simulink model "Modelo_Red_Mitigación_final"  (R2019b)
settings: Solver=VariableStepAuto  StartTime=0.0  StopTime=2.5  RelTol=1e-3
InitFcn:
  | Ts=20e-6;
undefined symbols (not defined in the file): D1, Delta, Ion, Lithium
libraries: powerlib x371, powerlib_meascontrol x286, simulink x50, simulink_extras x20, electricdrivelib x16
(part 2 of 11)

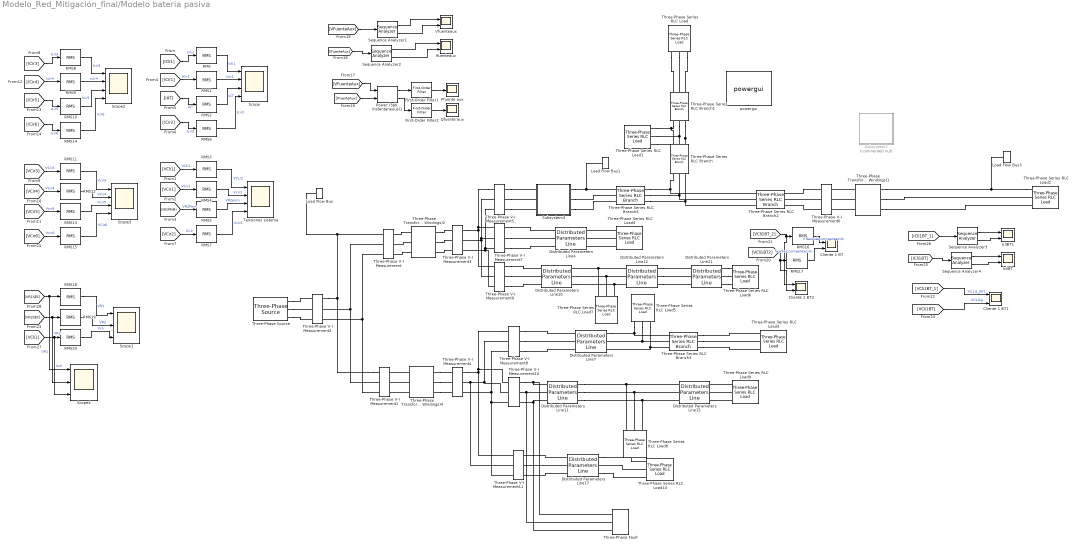
== system Modelo_Red_Mitigación_final/Modelo bateria pasiva ==
  Cliente 1 BT : Scope  NumInputPorts=2
  Cliente 1 BT1 : Scope  NumInputPorts=3
  Cliente 1 BT2 : Scope  NumInputPorts=2
  Distributed Parameters Line10 : powerlib/Elements/Distributed Parameters Line  Phases=3  Frequency=60  Resistance=[0.213 0.639]  Inductance=[0.78e-3 2.35e-3]  Capacitance=[15e-9 15e-9]  Length=3  x1=[-2e-05 -1.60744480727596e-09 32197.4628123978 -19329.1003175146;-1e-05 -1.62409816565211e-09 32270.1028326545 -19207.5816752185]  x2=[-2e-05 -1.47871788687323e-09 31710.064728457 -19350.950448235;-1e-05 -1.49515966537411e-09 31782.7905850735 -19231.2690938051]  x3=[-2e-05 7.10025507601476e-12 -137.606557855704 265.255923665208;-1e-05 7.2218880102072e-12 -138.605568913461 264.735275455604]  x4=[-2e-05 -1.17257744553877e-11 416.943661034857 -435.064418389001;-1e-05 -1.19305068231816e-11 418.580848520433 -433.489489927064]  x5=1.78115131305569e-05  V1=ones(3,3)  V2=ones(3,3)  I1=ones(3,3)  I2=ones(3,3)  nHarmo=1  Measurements=None
      settings: SourceProductName=Simscape Electrical
  Distributed Parameters Line11 : powerlib/Elements/Distributed Parameters Line  Phases=3  Frequency=60  Resistance=[0.269 0.807]  Inductance=[0.85e-3 2.56e-3]  Capacitance=[15e-9 15e-9]  Length=18  x1=[-0.00012 1.2995045318767e-09 31499.5304857104 -20459.5850295711;-0.00011 1.27437272136298e-09 31576.4372824135 -20340.6894905819;-0.0001 1.24922279919206e-09 31652.8953080482 -20221.5048653708;-9e-05 1.2240551228e-09 31728.9034759767 -20102.0328478151;-8e-05 1.19887004987519e-09 31804.4607059547 -19982.2751358768;-7e-05 1.17366793835327e-09 31879.5659241467 -19862.2334315779;-6e-05 1.14844914641202e-09 31954.2180631414 -19741.9094409767;-5e-05 1.1232140324663e-09 32028.4160619666 -19621.3048741436;-4e-05 1.09796295516295e-09 32102.1588661044 -19500.4214451364;-3e-05 1.07269627337565e-09 32175.4454275065 -19379.2608719761;-2e-05 1.04741434619989e-09 32248.2747046085 -19257.8248766228;-1e-05 1.02211753294781e-09 32320.6456623452 -19136.1151849507]  x2=[-0.00012 1.31071662041468e-09 29691.2836160795 -20133.8764409715;-0.00011 1.28874514200496e-09 29766.9753728354 -20021.8001304528;-0.0001 1.26675534767413e-09 29842.2440749819 -19909.4392658359;-9e-05 1.24474754994584e-09 29917.0886527841 -19796.7954440174;-8e-05 1.2227220615996e-09 29991.5080425349 -19683.8702659153;-7e-05 1.20067919566637e-09 30065.5011865701 -19570.6653364464;-6e-05 1.17861926542406e-09 30139.0670332832 -19457.1822645033;-5e-05 1.15654258439311e-09 30212.2045371409 -19343.4226629316;-4e-05 1.13444946633202e-09 30284.9126586972 -19229.3881485071;-3e-05 1.1123402252329e-09 30357.1903646088 -19115.0803419127;-2e-05 1.09021517531702e-09 30429.0366276495 -19000.5008677153;-1e-05 1.06807463103029e-09 30500.4504267249 -18885.6513543428]  x3=[-0.00012 -2.4045016954618e-11 9.2729752981831 123.36660820444;-0.00011 -2.40154356108507e-11 8.80782934902953 123.400689758634;-0.0001 -2.3985512954585e-11 8.34255822112473 123.43301751588;-9e-05 -2.39552494110883e-11 7.87716852700131 123.463591016726;-8e-05 -2.39246454104723e-11 7.41166688087696 123.492409826658;-7e-05 -2.38937013876877e-11 6.94605989856048 123.519473536094;-6e-05 -2.38624177825175e-11 6.4803541973577 123.5447817604;-5e-05 -2.38307950395711e-11 6.01455639597747 123.568334139891;-4e-05 -2.37988336082776e-11 5.54867311443761 123.590130339834;-3e-05 -2.37665339428797e-11 5.08271097397077 123.610170050458;-2e-05 -2.3733896502427e-11 4.61667659693038 123.628452986953;-1e-05 -2.370092175077e-11 4.15057660669652 123.64497888948]  x4=[-0.00012 3.0362726383601e-11 241.846087557241 -294.396448704912;-0.00011 3.02202025213524e-11 242.954214808817 -293.482620581595;-0.0001 3.00772491631334e-11 244.058889143221 -292.564621420615;-9e-05 2.99338683406276e-11 245.160094860585 -291.64246426877;-8e-05 2.97900620915938e-11 246.257816310337 -290.716162231956;-7e-05 2.96458324598374e-11 247.352037891427 -289.785728474975;-6e-05 2.95011814951804e-11 248.442744052543 -288.85117622135;-5e-05 2.93561112534334e-11 249.529919292337 -287.912518753138;-4e-05 2.92106237963656e-11 250.613548159642 -286.969769410738;-3e-05 2.90647211916758e-11 251.693615253694 -286.022941592705;-2e-05 2.89184055129629e-11 252.770105224347 -285.07204875556;-1e-05 2.87716788396966e-11 253.843002772297 -284.117104413593]  x5=0.000111541920370774  V1=ones(3,3)  V2=ones(3,3)  I1=ones(3,3)  I2=ones(3,3)  nHarmo=1  Measurements=None
      settings: SourceProductName=Simscape Electrical
  Distributed Parameters Line12 : powerlib/Elements/Distributed Parameters Line  Phases=3  Frequency=60  Resistance=[0.269 0.807]  Inductance=[0.85e-3 2.56e-3]  Capacitance=[15e-9 15e-9]  Length=6  x1=[-4e-05 -1.44392359072237e-09 0 0;-3e-05 -1.46041436185941e-09 31636.8882016302 -19470.3567828256;-2e-05 -1.47688437727574e-09 31710.064728457 -19350.950448235;-1e-05 -1.49333340289598e-09 31782.7905850735 -19231.2690938051]  x2=[-4e-05 -1.10440790101326e-09 0 0;-3e-05 -1.12027783273388e-09 30859.2103716388 -19384.6974111484;-2e-05 -1.13613184282675e-09 30932.0694972688 -19268.223454667;-1e-05 -1.1519697059713e-09 31004.489009723 -19151.47565408]  x3=[-4e-05 9.88842947250447e-12 0 0;-3e-05 1.00301842807399e-11 -40.5630647731756 176.429249490737;-2e-05 1.01717965378548e-11 -41.2278975531237 176.275076976319;-1e-05 1.03132642312256e-11 -41.8921443933894 176.11839920287]  x4=[-4e-05 -1.5358362467025e-11 0 0;-3e-05 -1.55737906928403e-11 301.110986467419 -339.882086337973;-2e-05 -1.57889975806172e-11 302.390168984157 -338.744512112845;-1e-05 -1.60039800717894e-11 303.665053867252 -337.602123578388]  x5=3.71806401235912e-05  V1=ones(3,3)  V2=ones(3,3)  I1=ones(3,3)  I2=ones(3,3)  nHarmo=1  Measurements=None
      settings: SourceProductName=Simscape Electrical
  Distributed Parameters Line15 : powerlib/Elements/Distributed Parameters Line  Phases=3  Frequency=60  Resistance=[0.269 0.807]  Inductance=[0.85e-3 2.56e-3]  Capacitance=[15e-9 15e-9]  Length=12  x1=[-8e-05 1.22092104036648e-09 0 0;-7e-05 1.19887583848136e-09 0 0;-6e-05 1.17681359791685e-09 0 0;-5e-05 1.15473463222624e-09 30212.2045371409 -19343.4226629316;-4e-05 1.13263925520049e-09 30284.9126586972 -19229.3881485071;-3e-05 1.11052778086381e-09 30357.1903646088 -19115.0803419127;-2e-05 1.08840052346922e-09 30429.0366276495 -19000.5008677153;-1e-05 1.06625779749401e-09 30500.4504267249 -18885.6513543428]  x2=[-8e-05 1.29624069193425e-09 0 0;-7e-05 1.2747888102258e-09 0 0;-6e-05 1.25331881094659e-09 0 0;-5e-05 1.23183099923286e-09 29831.7562384593 -19278.81027422;-4e-05 1.21032568047396e-09 29904.2234811319 -19166.210471837;-3e-05 1.18880316030808e-09 29976.2657185957 -19053.3382751787;-2e-05 1.16726374461788e-09 30047.8819269711 -18940.1952884088;-1e-05 1.14570773952611e-09 30119.0710884331 -18826.7831195396]  x3=[-8e-05 -1.86669864656838e-12 0 0;-7e-05 -1.87826047225921e-12 0 0;-6e-05 -1.88979560371118e-12 0 0;-5e-05 -1.90130387698456e-12 86.3804979588809 -15.5854425693707;-4e-05 -1.9127851285213e-12 86.4386397249209 -15.2596857835518;-3e-05 -1.9242391951474e-12 86.4955530065581 -14.9337121238205;-2e-05 -1.93566591407523e-12 86.5512369949287 -14.6075262229841;-1e-05 -1.9470651229058e-12 86.60569089864 -14.2811327168662]  x4=[-8e-05 7.83771383894334e-12 0 0;-7e-05 7.74849481913839e-12 0 0;-6e-05 7.65916567607072e-12 0 0;-5e-05 7.5697276793052e-12 162.002074810575 -147.043074965074;-4e-05 7.48018209995371e-12 162.555261626358 -146.431298074223;-3e-05 7.39053021065717e-12 163.106138172057 -145.817440070501;-2e-05 7.30077328556736e-12 163.654696618496 -145.201509678187;-1e-05 7.21091260032885e-12 164.200929169446 -144.583515651016]  x5=7.43612802471824e-05  V1=ones(3,3)  V2=ones(3,3)  I1=ones(3,3)  I2=ones(3,3)  nHarmo=1  Measurements=None
      settings: SourceProductName=Simscape Electrical
  Distributed Parameters Line17 : powerlib/Elements/Distributed Parameters Line  Phases=3  Frequency=60  Resistance=[0.213 0.639]  Inductance=[0.78e-3 2.35e-3]  Capacitance=[15e-9 15e-9]  Length=18  x1=[-0.00011 1.27437272136298e-09 31576.4372824135 -20340.6894905819;-0.0001 1.24922279919206e-09 31652.8953080482 -20221.5048653708;-9e-05 1.2240551228e-09 31728.9034759767 -20102.0328478151;-8e-05 1.19887004987519e-09 31804.4607059547 -19982.2751358768;-7e-05 1.17366793835326e-09 31879.5659241467 -19862.2334315779;-6e-05 1.14844914641202e-09 31954.2180631414 -19741.9094409767;-5e-05 1.1232140324663e-09 32028.4160619666 -19621.3048741436;-4e-05 1.09796295516295e-09 32102.1588661044 -19500.4214451364;-3e-05 1.07269627337565e-09 32175.4454275065 -19379.2608719761;-2e-05 1.04741434619989e-09 32248.2747046085 -19257.8248766228;-1e-05 1.02211753294781e-09 32320.6456623452 -19136.1151849507]  x2=[-0.00011 1.27963484134107e-09 30855.9731261018 -20386.4569187133;-0.0001 1.2554954697875e-09 30932.6088101621 -20269.9880477211;-9e-05 1.23133825486427e-09 31008.8048733818 -20153.2310953311;-8e-05 1.20716353989886e-09 31084.5602328461 -20036.1877209179;-7e-05 1.18297166846749e-09 31159.8738119037 -19918.859587927;-6e-05 1.15876298439019e-09 31234.7445401818 -19801.2483638508;-5e-05 1.13453783172596e-09 31309.1713536017 -19683.3557202053;-4e-05 1.11029655476783e-09 31383.1531943937 -19565.1833325057;-3e-05 1.08603949803802e-09 31456.689011112 -19446.7328802434;-2e-05 1.06176700628298e-09 31529.77775865 -19328.0060468613;-1e-05 1.03747942446855e-09 31602.4183982546 -19209.0045197307]  x3=[-0.00011 -6.91759926900062e-12 65.961633867162 -5.20882786214894;-0.0001 -6.9483977976633e-12 65.9808019086511 -4.96012193543562;-9e-05 -6.97909757421297e-12 65.9990322168963 -4.71134551441033;-8e-05 -7.00969816233783e-12 66.0163245328044 -4.4625021347367;-7e-05 -7.04019912713581e-12 66.0326786106134 -4.21359533302996;-6e-05 -7.07060003512067e-12 66.0480942178957 -3.96462864680672;-5e-05 -7.10090045422822e-12 66.0625711355614 -3.71560561443469;-4e-05 -7.13109995382243e-12 66.0761091578614 -3.46652977508236;-3e-05 -7.16119810470158e-12 66.0887080923904 -3.21740466866875;-2e-05 -7.1911944791043e-12 66.1003677600897 -2.96823383581305;-1e-05 -7.22108865071573e-12 66.1110879952497 -2.71902081778434]  x4=[-0.00011 1.38112426096876e-11 202.338595789282 -174.305940383178;-0.0001 1.37229379128099e-11 202.994274307245 -173.541905018119;-9e-05 1.36344381826086e-11 203.647067827242 -172.775403238454;-8e-05 1.35457446768608e-11 204.296967071631 -172.00644593787;-7e-05 1.34568586560976e-11 204.943962803905 -171.235044044951;-6e-05 1.33677813835861e-11 205.588045828824 -170.461208523027;-5e-05 1.32785141253114e-11 206.22920699254 -169.684950370013;-4e-05 1.3189058149959e-11 206.867437182737 -168.906280618256;-3e-05 1.30994147288962e-11 207.502727328748 -168.125210334376;-2e-05 1.30095851361545e-11 208.135068401696 -167.341750619111;-1e-05 1.29195706484112e-11 208.764451414614 -166.555912607158]  x5=0.000106869078783341  V1=ones(3,3)  V2=ones(3,3)  I1=ones(3,3)  I2=ones(3,3)  nHarmo=1  Measurements=None
      settings: SourceProductName=Simscape Electrical
  Distributed Parameters Line21 : powerlib/Elements/Distributed Parameters Line  Phases=3  Frequency=60  Resistance=[0.269 0.807]  Inductance=[0.85e-3 2.56e-3]  Capacitance=[15e-9 15e-9]  Length=3  x1=[-2e-05 -1.13612712838933e-09 30932.0694972688 -19268.223454667;-1e-05 -1.15196734873584e-09 31004.489009723 -19151.47565408]  x2=[-2e-05 -1.1316350606201e-09 30542.7078876874 -19225.7498451981;-1e-05 -1.1469927953962e-09 30614.9700456306 -19110.4702016429]  x3=[-2e-05 -2.73192015721216e-11 -43.7912955116792 177.913060929824;-1e-05 -2.72693838169427e-11 -44.461699175564 177.746707756943]  x4=[-2e-05 2.26989589517112e-11 301.055370571057 -339.730088442832;-1e-05 2.25858755556134e-11 302.3339804658 -338.592724964311]  x5=1.85903200617956e-05  V1=ones(3,3)  V2=ones(3,3)  I1=ones(3,3)  I2=ones(3,3)  nHarmo=1  Measurements=None
      settings: SourceProductName=Simscape Electrical
  Distributed Parameters Line4 : powerlib/Elements/Distributed Parameters Line  Phases=3  Frequency=60  Resistance=[0.213 0.639]  Inductance=[0.78e-3 2.35e-3]  Capacitance=[15e-9 15e-9]  Length=9  x1=[-6e-05 -1.54060529194429e-09 31902.337180431 -19812.4105819144;-5e-05 -1.55734860839913e-09 31976.8013303373 -19692.0010999493;-4e-05 -1.57406979148305e-09 32050.8110191159 -19571.3117510603;-3e-05 -1.59076860355102e-09 32124.3651949253 -19450.34425051;-2e-05 -1.60744480727596e-09 32197.4628123978 -19329.1003175146;-1e-05 -1.62409816565211e-09 32270.1028326545 -19207.5816752185]  x2=[-6e-05 -1.3573232705367e-09 31242.7818228174 -19858.7298296883;-5e-05 -1.37398741714429e-09 31317.4252786311 -19740.8064778034;-4e-05 -1.39063203634936e-09 31391.6236445103 -19622.602565362;-3e-05 -1.40725689159503e-09 31465.3758659321 -19504.1197723034;-2e-05 -1.42386174660529e-09 31538.6808947139 -19385.3597825304;-1e-05 -1.4404463653884e-09 31611.5376890293 -19266.3242838854]  x3=[-6e-05 6.90888111585168e-12 9.1850468948496 67.3502715851637;-5e-05 6.93155052985086e-12 8.93107768423515 67.3844197159407;-4e-05 6.95412143117399e-12 8.67698154323783 67.4176101649577;-3e-05 6.97659349903859e-12 8.42276208312623 67.4498424605051;-2e-05 6.99896641406685e-12 8.1684229169216 67.4811161444905;-1e-05 7.02123985829012e-12 7.91396765934648 67.5114307724457]  x4=[-6e-05 -1.16230620484614e-11 264.979509808266 -241.826806008708;-5e-05 -1.17319654356774e-11 265.889290256755 -240.826140710185;-4e-05 -1.18407020856958e-11 266.795291829882 -239.822052739133;-3e-05 -1.19492704531281e-11 267.697501651359 -238.814556365865;-2e-05 -1.20576689949774e-11 268.595906898788 -237.803665909133;-1e-05 -1.21658961706607e-11 269.490494803841 -236.789395735929]  x5=5.34345393916706e-05  V1=ones(3,3)  V2=ones(3,3)  I1=ones(3,3)  I2=ones(3,3)  nHarmo=1  Measurements=None
      settings: SourceProductName=Simscape Electrical
  Distributed Parameters Line7 : powerlib/Elements/Distributed Parameters Line  Phases=3  Frequency=60  Resistance=[0.213 0.639]  Inductance=[0.78e-3 2.35e-3]  Capacitance=[15e-9 15e-9]  Length=4.4  x1=[-3e-05 1.07267570152872e-09 0 0;-2e-05 1.04740063147284e-09 32248.2747046085 -19257.8248766228;-1e-05 1.02211067553556e-09 32320.6456623452 -19136.1151849507]  x2=[-3e-05 1.02319326387939e-09 0 0;-2e-05 9.98040734145155e-10 31944.5740855417 -19310.7767627753;-1e-05 9.72874020042916e-10 32017.1468248425 -19190.2116164699]  x3=[-3e-05 -1.12877964349124e-11 0 0;-2e-05 -1.13616672154719e-11 2.66918275739526 49.6416949019862;-1e-05 -1.14353765215912e-11 2.48201945236903 49.6514047008976]  x4=[-3e-05 1.056083567406e-11 0 0;-2e-05 1.05194622844416e-11 277.490011327236 -219.052715302666;-1e-05 1.04779393899792e-11 278.313846778869 -218.005048471382]  x5=2.61235525914834e-05  V1=ones(3,3)  V2=ones(3,3)  I1=ones(3,3)  I2=ones(3,3)  nHarmo=1  Measurements=None
      settings: SourceProductName=Simscape Electrical
  First-Order Filter1 : powerlib_meascontrol/Filters/First-Order Filter  FilterType=Lowpass  Tc=10e-3  Ts=0  Initialize=on  Vac_Init=[0, 0, 60]  Vdc_Init=0  PlotResponse=off  FreqRange="[0,  200,  1]"
      settings: SourceProductName=Simscape Electrical
  First-Order Filter2 : powerlib_meascontrol/Filters/First-Order Filter  FilterType=Lowpass  Tc=10e-3  Ts=0  Initialize=on  Vac_Init=[0, 0, 60]  Vdc_Init=0  PlotResponse=off  FreqRange="[0,  200,  1]"
      settings: SourceProductName=Simscape Electrical
  IcliBT : Scope  NumInputPorts=2
  IcliBT1 : Scope  NumInputPorts=2
  Ifuenteaux : Scope  NumInputPorts=2
  Load Flow Bus : powerlib/Measurements/Load Flow Bus  LConnTagsString=a  Phases=single  Connectors=on one side  ID=BUS_1  Vbase=115e3  Vref=1.05  Vangle=0  VLF=1  VLFb=1  VLFc=1  angleLF=0  angleLFb=0  angleLFc=0
      settings: SourceProductName=Simscape Electrical
  Load Flow Bus1 : powerlib/Measurements/Load Flow Bus  LConnTagsString=a  Phases=single  Connectors=on one side  ID=BUS_2  Vbase=115e3  Vref=0.9  Vangle=0  VLF=1  VLFb=1  VLFc=1  angleLF=0  angleLFb=0  angleLFc=0
      settings: SourceProductName=Simscape Electrical
  Load Flow Bus3 : powerlib/Measurements/Load Flow Bus  LConnTagsString=a  Phases=single  Connectors=on one side  ID=BUS_4  Vbase=440  Vref=1  Vangle=0  VLF=0.9785  VLFb=1  VLFc=1  angleLF=28.33  angleLFb=0  angleLFc=0
      settings: SourceProductName=Simscape Electrical
  "Pfuente aux " : Scope
  "Power (3ph, Instantaneous)1" : powerlib_meascontrol/Measurements/Power (3ph, Instantaneous)
      settings: SourceProductName=Simscape Electrical
  Qfuente aux : Scope
  RMS{,1..20} (21 alike) : powerlib_meascontrol/Measurements/RMS  TrueRMS=on  Freq=60  RMSInit=120  Ts=0
      settings: SourceProductName=Simscape Electrical
  Scope : Scope  NumInputPorts=4
  Scope1 : Scope  NumInputPorts=3
  Scope2 : Scope  NumInputPorts=4
  Scope3 : Scope  NumInputPorts=4
  Scope4 : Scope  NumInputPorts=3
  Sequence Analyzer{1..4} (4 alike) : powerlib_meascontrol/Measurements/Sequence Analyzer  Freq=60  n=1  seq=Positive Negative Zero  InInit=[1, 0]  Ts=0
      settings: SourceProductName=Simscape Electrical  SourceProductBaseCode=PS
  Subsystem2 : Subsystem  Commented=on
  Subsystem3 : Subsystem
  Tensiones sistema : Scope  NumInputPorts=4
  Three-Phase Series RLC Branch : powerlib/Elements/Three-Phase Series RLC Branch  LConnTagsString=A|B|C  RConnTagsString=A|B|C  BranchType=RL  Resistance=0.213  Inductance=0.78e-3  Capacitance=1e-6  Measurements=None
      settings: SourceProductName=Simscape Electrical
  Three-Phase Series RLC Branch1 : powerlib/Elements/Three-Phase Series RLC Branch  LConnTagsString=A|B|C  RConnTagsString=A|B|C  BranchType=RL  Resistance=0.213  Inductance=0.78e-3  Capacitance=1e-6  Measurements=None
      settings: SourceProductName=Simscape Electrical
  Three-Phase Series RLC Branch2 : powerlib/Elements/Three-Phase Series RLC Branch  LConnTagsString=A|B|C  RConnTagsString=A|B|C  BranchType=RL  Resistance=0.213*1.7  Inductance=0.78e-3*1.7  Capacitance=1e-6  Measurements=None
      settings: SourceProductName=Simscape Electrical
  Three-Phase Series RLC Branch3 : powerlib/Elements/Three-Phase Series RLC Branch  LConnTagsString=A|B|C  RConnTagsString=A|B|C  BranchType=RL  Resistance=0.213*2.2  Inductance=0.78e-3*2.2  Capacitance=1e-6  Measurements=None
      settings: SourceProductName=Simscape Electrical
  Three-Phase Series RLC Branch4 : powerlib/Elements/Three-Phase Series RLC Branch  LConnTagsString=A|B|C  RConnTagsString=A|B|C  BranchType=RL  Resistance=0.213*7  Inductance=0.78e-3*7  Capacitance=1e-6  Measurements=None
      settings: SourceProductName=Simscape Electrical
  Three-Phase Series RLC Load : powerlib/Elements/Three-Phase Series RLC Load  LConnTagsString=A|B|C  Configuration=Y (grounded)  NominalVoltage=34.5e3  Vabc=[1e3 1e3 1e3]  Vabcp=[1e3 1e3 1e3]  NominalFrequency=60  UnbalancedPower=off  ActivePower=0.5e6  InductivePower=0.1e6  CapacitivePower=0  Pabc=[10e3 9e3 11e3]  QLabc=[100 90 110]  QCabc=[100 90 110]  Pabcp=[10e3 9e3 11e3]  QLabcp=[100 90 110]  QCabcp=[100 90 110]  Measurements=None  LoadType=constant Z
      settings: SourceProductName=Simscape Electrical
  Three-Phase Series RLC Load1 : powerlib/Elements/Three-Phase Series RLC Load  LConnTagsString=A|B|C  Configuration=Y (grounded)  NominalVoltage=34.5e3  Vabc=[1e3 1e3 1e3]  Vabcp=[1e3 1e3 1e3]  NominalFrequency=60  UnbalancedPower=off  ActivePower=2.5e6  InductivePower=1e6  CapacitivePower=0  Pabc=[10e3 9e3 11e3]  QLabc=[100 90 110]  QCabc=[100 90 110]  Pabcp=[10e3 9e3 11e3]  QLabcp=[100 90 110]  QCabcp=[100 90 110]  Measurements=None  LoadType=constant Z
      settings: SourceProductName=Simscape Electrical
  Three-Phase Series RLC Load10 : powerlib/Elements/Three-Phase Series RLC Load  LConnTagsString=A|B|C  Configuration=Y (grounded)  NominalVoltage=34.5e3  Vabc=[1e3 1e3 1e3]  Vabcp=[1e3 1e3 1e3]  NominalFrequency=60  UnbalancedPower=off  ActivePower=3.4e6  InductivePower=1.1e6  CapacitivePower=0  Pabc=[10e3 9e3 11e3]  QLabc=[100 90 110]  QCabc=[100 90 110]  Pabcp=[10e3 9e3 11e3]  QLabcp=[100 90 110]  QCabcp=[100 90 110]  Measurements=None  LoadType=constant Z
      settings: SourceProductName=Simscape Electrical
  Three-Phase Series RLC Load2 : powerlib/Elements/Three-Phase Series RLC Load  LConnTagsString=A|B|C  Configuration=Y (grounded)  NominalVoltage=440  Vabc=[1e3 1e3 1e3]  Vabcp=[1e3 1e3 1e3]  NominalFrequency=60  UnbalancedPower=off  ActivePower=6.5e6  InductivePower=3e6  CapacitivePower=0  Pabc=[10e3 9e3 11e3]  QLabc=[100 90 110]  QCabc=[100 90 110]  Pabcp=[10e3 9e3 11e3]  QLabcp=[100 90 110]  QCabcp=[100 90 110]  Measurements=None  LoadType=constant Z
      settings: SourceProductName=Simscape Electrical
  Three-Phase Series RLC Load3 : powerlib/Elements/Three-Phase Series RLC Load  LConnTagsString=A|B|C  Configuration=Y (grounded)  NominalVoltage=34.5e3  Vabc=[1e3 1e3 1e3]  Vabcp=[1e3 1e3 1e3]  NominalFrequency=60  UnbalancedPower=off  ActivePower=3e6  InductivePower=0.7e6  CapacitivePower=0  Pabc=[10e3 9e3 11e3]  QLabc=[100 90 110]  QCabc=[100 90 110]  Pabcp=[10e3 9e3 11e3]  QLabcp=[100 90 110]  QCabcp=[100 90 110]  Measurements=None  LoadType=constant Z
      settings: SourceProductName=Simscape Electrical
  Three-Phase Series RLC Load4 : powerlib/Elements/Three-Phase Series RLC Load  LConnTagsString=A|B|C  Configuration=Y (grounded)  NominalVoltage=34.5e3  Vabc=[1e3 1e3 1e3]  Vabcp=[1e3 1e3 1e3]  NominalFrequency=60  UnbalancedPower=off  ActivePower=6.2e6  InductivePower=2e6  CapacitivePower=0  Pabc=[10e3 9e3 11e3]  QLabc=[100 90 110]  QCabc=[100 90 110]  Pabcp=[10e3 9e3 11e3]  QLabcp=[100 90 110]  QCabcp=[100 90 110]  Measurements=None  LoadType=constant Z
      settings: SourceProductName=Simscape Electrical
  Three-Phase Series RLC Load5 : powerlib/Elements/Three-Phase Series RLC Load  LConnTagsString=A|B|C  Configuration=Y (grounded)  NominalVoltage=34.5e3  Vabc=[1e3 1e3 1e3]  Vabcp=[1e3 1e3 1e3]  NominalFrequency=60  UnbalancedPower=off  ActivePower=3e6  InductivePower=0.7e6  CapacitivePower=0  Pabc=[10e3 9e3 11e3]  QLabc=[100 90 110]  QCabc=[100 90 110]  Pabcp=[10e3 9e3 11e3]  QLabcp=[100 90 110]  QCabcp=[100 90 110]  Measurements=None  LoadType=constant Z
      settings: SourceProductName=Simscape Electrical
  Three-Phase Series RLC Load6 : powerlib/Elements/Three-Phase Series RLC Load  LConnTagsString=A|B|C  Configuration=Y (grounded)  NominalVoltage=34.5e3  Vabc=[1e3 1e3 1e3]  Vabcp=[1e3 1e3 1e3]  NominalFrequency=60  UnbalancedPower=off  ActivePower=9.4e6  InductivePower=4.2e6  CapacitivePower=0  Pabc=[10e3 9e3 11e3]  QLabc=[100 90 110]  QCabc=[100 90 110]  Pabcp=[10e3 9e3 11e3]  QLabcp=[100 90 110]  QCabcp=[100 90 110]  Measurements=None  LoadType=constant Z
      settings: SourceProductName=Simscape Electrical
  Three-Phase Series RLC Load7 : powerlib/Elements/Three-Phase Series RLC Load  LConnTagsString=A|B|C  Configuration=Y (grounded)  NominalVoltage=34.5e3  Vabc=[1e3 1e3 1e3]  Vabcp=[1e3 1e3 1e3]  NominalFrequency=60  UnbalancedPower=off  ActivePower=4.4e6  InductivePower=0.8e6  CapacitivePower=0  Pabc=[10e3 9e3 11e3]  QLabc=[100 90 110]  QCabc=[100 90 110]  Pabcp=[10e3 9e3 11e3]  QLabcp=[100 90 110]  QCabcp=[100 90 110]  Measurements=None  LoadType=constant Z
      settings: SourceProductName=Simscape Electrical
  Three-Phase Series RLC Load8 : powerlib/Elements/Three-Phase Series RLC Load  LConnTagsString=A|B|C  Configuration=Y (grounded)  NominalVoltage=34.5e3  Vabc=[1e3 1e3 1e3]  Vabcp=[1e3 1e3 1e3]  NominalFrequency=60  UnbalancedPower=off  ActivePower=5e6  InductivePower=2.5e6  CapacitivePower=0  Pabc=[10e3 9e3 11e3]  QLabc=[100 90 110]  QCabc=[100 90 110]  Pabcp=[10e3 9e3 11e3]  QLabcp=[100 90 110]  QCabcp=[100 90 110]  Measurements=None  LoadType=constant Z
      settings: SourceProductName=Simscape Electrical
  Three-Phase Series RLC Load9 : powerlib/Elements/Three-Phase Series RLC Load  LConnTagsString=A|B|C  Configuration=Y (grounded)  NominalVoltage=34.5e3  Vabc=[1e3 1e3 1e3]  Vabcp=[1e3 1e3 1e3]  NominalFrequency=60  UnbalancedPower=off  ActivePower=2.3e6  InductivePower=1.2e6  CapacitivePower=0  Pabc=[10e3 9e3 11e3]  QLabc=[100 90 110]  QCabc=[100 90 110]  Pabcp=[10e3 9e3 11e3]  QLabcp=[100 90 110]  QCabcp=[100 90 110]  Measurements=None  LoadType=constant Z
      settings: SourceProductName=Simscape Electrical
  Three-Phase V-I Measurement : powerlib/Measurements/Three-Phase V-I Measurement  VoltageMeasurement=phase-to-ground  SetLabelV=on  LabelV=VR2PRIM  Vpu=off  VpuLL=off  CurrentMeasurement=yes  SetLabelI=on  LabelI=IR2PRIM  Ipu=off  Pbase=100e6  Vbase=500e3  OutputType=Complex  PhasorSimulation=off  PSBequivalent=0
      settings: SourceProductName=Simscape Electrical
  Three-Phase V-I Measurement1 : powerlib/Measurements/Three-Phase V-I Measurement  VoltageMeasurement=phase-to-ground  SetLabelV=on  LabelV=VR1PRIM  Vpu=off  VpuLL=off  CurrentMeasurement=yes  SetLabelI=on  LabelI=IR1PRIM  Ipu=off  Pbase=100e6  Vbase=500e3  OutputType=Complex  PhasorSimulation=off  PSBequivalent=0
      settings: SourceProductName=Simscape Electrical
  Three-Phase V-I Measurement10 : powerlib/Measurements/Three-Phase V-I Measurement  VoltageMeasurement=phase-to-ground  SetLabelV=on  LabelV=VCir5  Vpu=off  VpuLL=off  CurrentMeasurement=yes  SetLabelI=on  LabelI=ICir5  Ipu=off  Pbase=100e6  Vbase=500e3  OutputType=Complex  PhasorSimulation=off  PSBequivalent=0
      settings: SourceProductName=Simscape Electrical
  Three-Phase V-I Measurement11 : powerlib/Measurements/Three-Phase V-I Measurement  VoltageMeasurement=phase-to-ground  SetLabelV=on  LabelV=VCir6  Vpu=off  VpuLL=off  CurrentMeasurement=yes  SetLabelI=on  LabelI=ICir6  Ipu=off  Pbase=100e6  Vbase=500e3  OutputType=Complex  PhasorSimulation=off  PSBequivalent=0
      settings: SourceProductName=Simscape Electrical
  Three-Phase V-I Measurement2 : powerlib/Measurements/Three-Phase V-I Measurement  VoltageMeasurement=phase-to-ground  SetLabelV=on  LabelV=VAT  Vpu=off  VpuLL=off  CurrentMeasurement=yes  SetLabelI=on  LabelI=IAT  Ipu=off  Pbase=100e6  Vbase=500e3  OutputType=Complex  PhasorSimulation=off  PSBequivalent=0
      settings: SourceProductName=Simscape Electrical
  Three-Phase V-I Measurement3 : powerlib/Measurements/Three-Phase V-I Measurement  VoltageMeasurement=phase-to-ground  SetLabelV=on  LabelV=VR2SEC  Vpu=off  VpuLL=off  CurrentMeasurement=yes  SetLabelI=on  LabelI=IR2SEC  Ipu=off  Pbase=100e6  Vbase=500e3  OutputType=Complex  PhasorSimulation=off  PSBequivalent=0
      settings: SourceProductName=Simscape Electrical
  Three-Phase V-I Measurement4 : powerlib/Measurements/Three-Phase V-I Measurement  VoltageMeasurement=phase-to-ground  SetLabelV=on  LabelV=VR1SEC  Vpu=off  VpuLL=off  CurrentMeasurement=yes  SetLabelI=on  LabelI=IR1SEC  Ipu=off  Pbase=100e6  Vbase=500e3  OutputType=Complex  PhasorSimulation=off  PSBequivalent=0
      settings: SourceProductName=Simscape Electrical
  Three-Phase V-I Measurement5 : powerlib/Measurements/Three-Phase V-I Measurement  VoltageMeasurement=phase-to-ground  SetLabelV=on  LabelV=VCir1  Vpu=off  VpuLL=off  CurrentMeasurement=yes  SetLabelI=on  LabelI=ICir1  Ipu=off  Pbase=100e6  Vbase=500e3  OutputType=Complex  PhasorSimulation=off  PSBequivalent=0
      settings: SourceProductName=Simscape Electrical
  Three-Phase V-I Measurement6 : powerlib/Measurements/Three-Phase V-I Measurement  VoltageMeasurement=phase-to-ground  SetLabelV=on  LabelV=VCli1  Vpu=off  VpuLL=off  CurrentMeasurement=yes  SetLabelI=on  LabelI=ICli1  Ipu=off  Pbase=100e6  Vbase=500e3  OutputType=Complex  PhasorSimulation=off  PSBequivalent=0
      settings: SourceProductName=Simscape Electrical
  Three-Phase V-I Measurement7 : powerlib/Measurements/Three-Phase V-I Measurement  VoltageMeasurement=phase-to-ground  SetLabelV=on  LabelV=VCir2  Vpu=off  VpuLL=off  CurrentMeasurement=yes  SetLabelI=on  LabelI=ICir2  Ipu=off  Pbase=100e6  Vbase=500e3  OutputType=Complex  PhasorSimulation=off  PSBequivalent=0
      settings: SourceProductName=Simscape Electrical
  Three-Phase V-I Measurement8 : powerlib/Measurements/Three-Phase V-I Measurement  VoltageMeasurement=phase-to-ground  SetLabelV=on  LabelV=VCir4  Vpu=off  VpuLL=off  CurrentMeasurement=yes  SetLabelI=on  LabelI=ICir4  Ipu=off  Pbase=100e6  Vbase=500e3  OutputType=Complex  PhasorSimulation=off  PSBequivalent=0
      settings: SourceProductName=Simscape Electrical
  Three-Phase V-I Measurement9 : powerlib/Measurements/Three-Phase V-I Measurement  VoltageMeasurement=phase-to-ground  SetLabelV=on  LabelV=VCir3  Vpu=off  VpuLL=off  CurrentMeasurement=yes  SetLabelI=on  LabelI=ICir3  Ipu=off  Pbase=100e6  Vbase=500e3  OutputType=Complex  PhasorSimulation=off  PSBequivalent=0
      settings: SourceProductName=Simscape Electrical
  Three-Phase Fault : powerlib/Elements/Three-Phase Fault  InitialStates=0  FaultA=on  FaultB=on  FaultC=on  GroundFault=off  SwitchTimes=[0.1,0.8,0.9,1.6,1.7,2.4]  External=off  SwitchStatus=NaN  FaultResistance=0.3  GroundResistance=0.01  SnubberResistance=1e6  SnubberCapacitance=inf  Measurements=None
      settings: SourceProductName=Simscape Electrical
  Three-Phase Source : powerlib/Electrical Sources/Three-Phase Source  InternalConnection=Yg  VoltagePhases=off  Voltage=(115000)*1.39942  PhaseAngle=16.7311  Voltage_phases=[25e3 25e3 25e3]/sqrt(3)  PhaseAngles_phases=[0 -120 +120]  Frequency=60  NonIdealSource=on  SpecifyImpedance=on  Resistance=0.8929  Inductance=16.58e-3  ShortCircuitLevel=100e6  BaseVoltage=115e3  XRratio=5.946  BusType=swing  Pref=10e3  Qref=0  Prefabc=[10e3, 10e3, 10e3]  Qrefabc=[0, 0, 0]  Qmin=-inf  Qmax=inf
      settings: SourceProductName=Simscape Electrical
  Three-Phase Transformer Inductance Matrix Type (Two Windings)1 : powerlib/Elements/Three-Phase Transformer Inductance Matrix Type (Two Windings)  CoreType=Three-limb or five-limb core  Winding1Connection=Yg  Winding2Connection=Yg  AutoTransformer=off  Measurements=None  NominalPower=[10e6, 60]  VLLnom=[34.5e3, 440]  WindingResistances=[0.01, 0.01]  NoLoadIexcPos=2  NoLoadPlossPos=1000  ShortCircuitReactancePos=0.06  ShortCircuitReactancePosAuto=0.06  NoLoadIexcZero=100  NoLoadPlossZero=500000  ShortCircuitReactanceZero=0.03  ShortCircuitReactanceZeroAuto=0.03
      settings: SourceProductName=Simscape Electrical  SourceProductBaseCode=PS
  Three-Phase Transformer Inductance Matrix Type (Two Windings)2 : powerlib/Elements/Three-Phase Transformer Inductance Matrix Type (Two Windings)  CoreType=Three single-phase cores  Winding1Connection=Delta (D1)  Winding2Connection=Y  AutoTransformer=off  Measurements=None  NominalPower=[40e6, 60]  VLLnom=[115e3, 34.5e3]  WindingResistances=[0.006, 0.006]  NoLoadIexcPos=2  NoLoadPlossPos=16600  ShortCircuitReactancePos=0.1056  ShortCircuitReactancePosAuto=0.06  NoLoadIexcZero=100  NoLoadPlossZero=500000  ShortCircuitReactanceZero=0.1056  ShortCircuitReactanceZeroAuto=0.03
      settings: SourceProductName=Simscape Electrical  SourceProductBaseCode=PS
  Three-Phase Transformer Inductance Matrix Type (Two Windings)4 : powerlib/Elements/Three-Phase Transformer Inductance Matrix Type (Two Windings)  CoreType=Three single-phase cores  Winding1Connection=Delta (D1)  Winding2Connection=Y  AutoTransformer=off  Measurements=None  NominalPower=[30e6, 60]  VLLnom=[115e3, 34.5e3]  WindingResistances=[0.006, 0.006]  NoLoadIexcPos=2  NoLoadPlossPos=14300  ShortCircuitReactancePos=0.0912  ShortCircuitReactancePosAuto=0.06  NoLoadIexcZero=100  NoLoadPlossZero=500000  ShortCircuitReactanceZero=0.0912  ShortCircuitReactanceZeroAuto=0.03
      settings: SourceProductName=Simscape Electrical  SourceProductBaseCode=PS
  Vfuenteaux : Scope  NumInputPorts=2
  powergui : powerlib/powergui  Priority=1  SimulationMode=Discrete  SampleTime=10e-6  frequency=60  Iterations=50  frequencyindice=0  Pbase=100e6  ErrMax=0.0001  UnitsV=kV  UnitsW=MW  buscounter=0  FunctionMessages=off  echomessages=off  EnableUseOfTLC=off  CurrentSourceSwitches=off  DisableSnubberDevices=off  DisableRonSwitches=off  DisableVfSwitches=off  DisplayEquations=off  AutomaticDiscreteSolvers=off  SolverType=Tustin/Backward Euler (TBE)  Interpol=off  ExternalGateDelay=off  methode=off  Ts=100  x0status=blocks  SPID=on  SwTol=0  HookPort=off  NonlinearTolerance=1e-4  nMaxIteration=100  ContinueOnMaxIteration=off  RestoreLinks=warning  ResistiveCurrentMeasurement=off  Frange=[0:2:500]  Ylog=off  Xlog=on  ShowGrid=off  save=off  variable=ZData  structure=0  ZoomFFT=off  StartTime=0.0  cycles=1  DisplayStyle=1  fundamental=60  FreqAxis=off  MaxFrequency=1000  frequencyindicesteady=1  RmsSteady=1  display=off
      settings: SourceProductName=Simscape Electrical
  wires:
  [VCli1] -> RMS20/1, Scope4/3  "Vcli"
  RMS19/1 -> Scope1/2  "VR2"
  RMS18/1 -> Scope1/1  "VR1"
  [VR2SEC] -> RMS19/1, Scope4/2  "VR2"
  [VR1SEC] -> RMS18/1, Scope4/1  "VR1"
  [VCli1BT_2] -> RMS16/1, Cliente 1 BT2/1
  Sequence Analyzer1/1 -> Vfuenteaux/1
  Sequence Analyzer2/2 -> Ifuenteaux/2
  [IFuenteAux] -> Sequence Analyzer2/1
  RMS8/1 -> Scope2/1  "Icir3"
  "Power (3ph, Instantaneous)1"/1 -> First-Order Filter1/1
  RMS11/1 -> Scope3/1  "Vcir3"
  [IFuenteAux] -> "Power (3ph, Instantaneous)1"/2
  RMS10/1 -> Scope2/3  "Icir5"
  RMS12/1 -> Scope3/2  "VCir4"
  [VFuenteAux] -> "Power (3ph, Instantaneous)1"/1
  [ICir4] -> RMS9/1  "Icir4"
  [VCir4] -> RMS12/1  "VCir4"
  [ICir3] -> RMS8/1  "Icir3"
  RMS15/1 -> Scope3/4  "VCir6"
  RMS2/1 -> Scope/3  "IAT"
  [IAT] -> RMS2/1  "IAT"
  [ICir6] -> RMS14/1  "Icir6"
  [VR2PRIM] -> RMS5/1  "VR2Prim"
  RMS4/1 -> Tensiones sistema/2  "Vcir1"
  [VCir1] -> RMS4/1  "VCir1"
  [ICli1] -> RMS/1  "Icli1"
  RMS/1 -> Scope/1  "Icli1"
  RMS6/1 -> Scope/4  "Icir2"
  First-Order Filter2/1 -> Qfuente aux/1
  RMS14/1 -> Scope2/4  "Icir6"
  [ICli1BT_1] -> Sequence Analyzer3/1
  [VCir2] -> RMS7/1  "Cir2"
  RMS16/1 -> Cliente 1 BT/1  "V después compensación"
  RMS17/1 -> Cliente 1 BT/2  "V antes compensación"
  [VCli1BT_1] -> Cliente 1 BT1/1  "VCLI1_BT1"
  Sequence Analyzer2/1 -> Ifuenteaux/1
  Sequence Analyzer3/2 -> IcliBT1/2
  [VCli1BT] -> Cliente 1 BT1/3  "VCLI1g"
  RMS3/1 -> Tensiones sistema/1  "VCLI1"
  First-Order Filter1/1 -> "Pfuente aux "/1
  [ICli1BT] -> Sequence Analyzer4/1
  [VCir6] -> RMS15/1  "Vcir6"
  [ICir1] -> RMS1/1  "ICir1"
  [VCli1BT2] -> RMS17/1, Cliente 1 BT2/2
  [VCir5] -> RMS13/1  "Vcir5"
  [VFuenteAux] -> Sequence Analyzer1/1
  [VCir3] -> RMS11/1  "VCir3"
  RMS9/1 -> Scope2/2  "Icir4"
  Sequence Analyzer4/1 -> IcliBT/1
  Sequence Analyzer3/1 -> IcliBT1/1
  RMS7/1 -> Tensiones sistema/4  "Vcir2"
  [ICir2] -> RMS6/1  "Icir2"
  Sequence Analyzer1/2 -> Vfuenteaux/2
  [ICir5] -> RMS10/1  "Icir5"
  RMS13/1 -> Scope3/3  "VCir5"
  "Power (3ph, Instantaneous)1"/2 -> First-Order Filter2/1
  [VCli1] -> RMS3/1  "VCli1"
  RMS5/1 -> Tensiones sistema/3  "VR2prim"
  Sequence Analyzer4/2 -> IcliBT/2
  RMS1/1 -> Scope/2  "Icir1"
  RMS20/1 -> Scope1/3  "Vcli"
  connections:
  Distributed Parameters Line21/RConn1 -- Three-Phase Series RLC Load6/LConn1
  Three-Phase Series RLC Load4/LConn1 -- Distributed Parameters Line4/RConn1
  Three-Phase Transformer Inductance Matrix Type (Two Windings)1/LConn3 -- Three-Phase V-I Measurement6/RConn3
  Three-Phase Series RLC Load10/LConn2 -- Distributed Parameters Line17/RConn2
  Three-Phase V-I Measurement7/RConn3 -- Distributed Parameters Line4/LConn3
  Three-Phase Transformer Inductance Matrix Type (Two Windings)2/LConn1 -- Three-Phase V-I Measurement/RConn1
  Three-Phase Series RLC Load4/LConn2 -- Distributed Parameters Line4/RConn2
  Three-Phase Series RLC Load4/LConn3 -- Distributed Parameters Line4/RConn3
  Three-Phase Series RLC Load9/LConn1 -- Distributed Parameters Line15/RConn1
  Distributed Parameters Line17/RConn1 -- Three-Phase Series RLC Load10/LConn1
  Three-Phase Series RLC Load/LConn3 -- Three-Phase Series RLC Branch1/RConn3
  Three-Phase V-I Measurement4/RConn2 -- Three-Phase V-I Measurement11/LConn2 -- Three-Phase V-I Measurement10/LConn2 -- Three-Phase V-I Measurement8/LConn2
  Three-Phase Transformer Inductance Matrix Type (Two Windings)2/LConn2 -- Three-Phase V-I Measurement/RConn2
  Three-Phase Transformer Inductance Matrix Type (Two Windings)2/LConn3 -- Three-Phase V-I Measurement/RConn3
  Three-Phase Series RLC Branch3/LConn3 -- Distributed Parameters Line7/RConn3 -- Three-Phase Series RLC Load5/LConn3
  Distributed Parameters Line21/RConn3 -- Three-Phase Series RLC Load6/LConn3
  Distributed Parameters Line12/RConn2 -- Distributed Parameters Line21/LConn2
  Distributed Parameters Line12/RConn1 -- Distributed Parameters Line21/LConn1
  Three-Phase Series RLC Load7/LConn1 -- Distributed Parameters Line10/RConn1 -- Distributed Parameters Line12/LConn1
  Distributed Parameters Line11/LConn2 -- Three-Phase Fault/LConn2 -- Three-Phase V-I Measurement10/RConn2
  Three-Phase V-I Measurement10/RConn1 -- Three-Phase Fault/LConn1 -- Distributed Parameters Line11/LConn1
  Three-Phase V-I Measurement8/RConn2 -- Distributed Parameters Line7/LConn2
  Distributed Parameters Line17/LConn2 -- Three-Phase V-I Measurement11/RConn2
  Three-Phase V-I Measurement9/RConn2 -- Distributed Parameters Line10/LConn2
  Three-Phase V-I Measurement4/RConn3 -- Three-Phase V-I Measurement11/LConn3 -- Three-Phase V-I Measurement10/LConn3 -- Three-Phase V-I Measurement8/LConn3
  Distributed Parameters Line17/RConn3 -- Three-Phase Series RLC Load10/LConn3
  Distributed Parameters Line17/LConn3 -- Three-Phase V-I Measurement11/RConn3
  Three-Phase V-I Measurement9/RConn1 -- Distributed Parameters Line10/LConn1
  Three-Phase Series RLC Load/LConn2 -- Three-Phase Series RLC Branch1/RConn2
  Three-Phase V-I Measurement8/RConn1 -- Distributed Parameters Line7/LConn1
  Three-Phase Series RLC Load5/LConn2 -- Three-Phase Series RLC Branch3/LConn2 -- Distributed Parameters Line7/RConn2
  Three-Phase V-I Measurement7/RConn2 -- Distributed Parameters Line4/LConn2
  Three-Phase V-I Measurement2/RConn3 -- Three-Phase V-I Measurement1/LConn3 -- Three-Phase V-I Measurement/LConn3
  Three-Phase V-I Measurement7/RConn1 -- Distributed Parameters Line4/LConn1
  Distributed Parameters Line11/RConn1 -- Distributed Parameters Line15/LConn1 -- Three-Phase Series RLC Load8/LConn1
  Three-Phase V-I Measurement6/LConn3 -- Three-Phase Series RLC Branch2/RConn3
  Three-Phase Transformer Inductance Matrix Type (Two Windings)1/LConn1 -- Three-Phase V-I Measurement6/RConn1
  Three-Phase Series RLC Load/LConn1 -- Three-Phase Series RLC Branch1/RConn1
  Three-Phase Transformer Inductance Matrix Type (Two Windings)1/LConn2 -- Three-Phase V-I Measurement6/RConn2
  Three-Phase V-I Measurement6/LConn1 -- Three-Phase Series RLC Branch2/RConn1
  Three-Phase Series RLC Branch/RConn3 -- Three-Phase Series RLC Branch1/LConn3 -- Three-Phase Series RLC Load1/LConn3
  Three-Phase Series RLC Branch/RConn2 -- Three-Phase Series RLC Branch1/LConn2 -- Three-Phase Series RLC Load1/LConn2
  Three-Phase Series RLC Branch2/LConn2 -- Three-Phase Series RLC Branch4/RConn2 -- Three-Phase Series RLC Branch/LConn2
  Three-Phase Transformer Inductance Matrix Type (Two Windings)4/LConn3 -- Three-Phase V-I Measurement1/RConn3
  Three-Phase Series RLC Load9/LConn2 -- Distributed Parameters Line15/RConn2
  Three-Phase Transformer Inductance Matrix Type (Two Windings)4/LConn2 -- Three-Phase V-I Measurement1/RConn2
  Three-Phase Transformer Inductance Matrix Type (Two Windings)2/RConn2 -- Three-Phase V-I Measurement3/LConn2
  Distributed Parameters Line21/RConn2 -- Three-Phase Series RLC Load6/LConn2
  Three-Phase V-I Measurement8/LConn1 -- Three-Phase V-I Measurement10/LConn1 -- Three-Phase V-I Measurement11/LConn1 -- Three-Phase V-I Measurement4/RConn1
  Three-Phase Source/RConn3 -- Three-Phase V-I Measurement2/LConn3
  Three-Phase Source/RConn2 -- Three-Phase V-I Measurement2/LConn2
  Three-Phase V-I Measurement1/LConn1 -- Three-Phase V-I Measurement/LConn1 -- Load Flow Bus/LConn1 -- Three-Phase V-I Measurement2/RConn1
  Three-Phase Series RLC Load7/LConn3 -- Distributed Parameters Line10/RConn3 -- Distributed Parameters Line12/LConn3
  Three-Phase Series RLC Branch/RConn1 -- Three-Phase Series RLC Branch1/LConn1 -- Three-Phase Series RLC Load1/LConn1
  Distributed Parameters Line12/RConn3 -- Distributed Parameters Line21/LConn3
  Three-Phase V-I Measurement3/LConn3 -- Three-Phase Transformer Inductance Matrix Type (Two Windings)2/RConn3
  Three-Phase Transformer Inductance Matrix Type (Two Windings)4/RConn3 -- Three-Phase V-I Measurement4/LConn3
  Three-Phase Series RLC Branch2/LConn1 -- Three-Phase Series RLC Branch/LConn1 -- Three-Phase Series RLC Branch4/RConn1
  Three-Phase Transformer Inductance Matrix Type (Two Windings)4/RConn2 -- Three-Phase V-I Measurement4/LConn2
  Subsystem3/RConn1 -- Load Flow Bus1/LConn1 -- Three-Phase Series RLC Branch4/LConn1
  Three-Phase V-I Measurement3/RConn3 -- Three-Phase V-I Measurement9/LConn3 -- Three-Phase V-I Measurement7/LConn3 -- Three-Phase V-I Measurement5/LConn3
  Three-Phase V-I Measurement5/RConn2 -- Subsystem3/LConn2
  Three-Phase Transformer Inductance Matrix Type (Two Windings)4/LConn1 -- Three-Phase V-I Measurement1/RConn1
  Three-Phase Series RLC Branch3/RConn3 -- Three-Phase Series RLC Load3/LConn3
  Three-Phase Series RLC Load2/LConn1 -- Three-Phase Transformer Inductance Matrix Type (Two Windings)1/RConn1 -- Load Flow Bus3/LConn1
  Three-Phase Series RLC Branch3/RConn1 -- Three-Phase Series RLC Load3/LConn1
  Three-Phase V-I Measurement5/LConn1 -- Three-Phase V-I Measurement7/LConn1 -- Three-Phase V-I Measurement9/LConn1 -- Three-Phase V-I Measurement3/RConn1
  Three-Phase V-I Measurement9/RConn3 -- Distributed Parameters Line10/LConn3
  Distributed Parameters Line11/RConn2 -- Distributed Parameters Line15/LConn2 -- Three-Phase Series RLC Load8/LConn2
  Three-Phase V-I Measurement8/RConn3 -- Distributed Parameters Line7/LConn3
  Three-Phase Transformer Inductance Matrix Type (Two Windings)4/RConn1 -- Three-Phase V-I Measurement4/LConn1
  Distributed Parameters Line17/LConn1 -- Three-Phase V-I Measurement11/RConn1
  Three-Phase V-I Measurement5/RConn1 -- Subsystem3/LConn1
  Subsystem3/RConn2 -- Three-Phase Series RLC Branch4/LConn2
  Three-Phase Series RLC Load5/LConn1 -- Three-Phase Series RLC Branch3/LConn1 -- Distributed Parameters Line7/RConn1
  Three-Phase Series RLC Branch4/RConn3 -- Three-Phase Series RLC Branch2/LConn3 -- Three-Phase Series RLC Branch/LConn3
  Three-Phase V-I Measurement2/RConn2 -- Three-Phase V-I Measurement1/LConn2 -- Three-Phase V-I Measurement/LConn2
  Three-Phase Transformer Inductance Matrix Type (Two Windings)1/RConn3 -- Three-Phase Series RLC Load2/LConn3
  Three-Phase Series RLC Branch3/RConn2 -- Three-Phase Series RLC Load3/LConn2
  Three-Phase V-I Measurement6/LConn2 -- Three-Phase Series RLC Branch2/RConn2
  Subsystem3/RConn3 -- Three-Phase Series RLC Branch4/LConn3
  Three-Phase Source/RConn1 -- Three-Phase V-I Measurement2/LConn1
  Three-Phase Series RLC Load7/LConn2 -- Distributed Parameters Line10/RConn2 -- Distributed Parameters Line12/LConn2
  Three-Phase V-I Measurement7/LConn2 -- Three-Phase V-I Measurement9/LConn2 -- Three-Phase V-I Measurement3/RConn2 -- Three-Phase V-I Measurement5/LConn2
  Three-Phase Series RLC Load8/LConn3 -- Distributed Parameters Line11/RConn3 -- Distributed Parameters Line15/LConn3
  Three-Phase V-I Measurement5/RConn3 -- Subsystem3/LConn3
  Three-Phase Transformer Inductance Matrix Type (Two Windings)2/RConn1 -- Three-Phase V-I Measurement3/LConn1
  Three-Phase V-I Measurement10/RConn3 -- Three-Phase Fault/LConn3 -- Distributed Parameters Line11/LConn3
  Three-Phase Transformer Inductance Matrix Type (Two Windings)1/RConn2 -- Three-Phase Series RLC Load2/LConn2
  Three-Phase Series RLC Load9/LConn3 -- Distributed Parameters Line15/RConn3
